simulink model "dodatkowa"  (R2022b)
settings: Solver=VariableStepAuto  StartTime=0.0  StopTime=10.0  RelTol=1e-3
values from neighbouring files (symbols this model uses):
  A = [0,       1,             0, 0 ... (first row only)    [dodatkowe.m]
  b = [0, 1/M, 0, 1/(M*L)]'    [dodatkowe.m]
  C = [1,0,0,0 ... (first row only)    [dodatkowe.m]
  D = [0, 0, 0,0]'    [dodatkowe.m]
  K = lqr(system, Q, R)    [dodatkowe.m]
  x0 = [0, 0, 0, 0]'    [dodatkowe.m]
  Y = [y, 0, 0, 0]'    [dodatkowe.m]
libraries: eeLuenbergerObserver x1
settings Model: Creator=student  LastModifiedBy=asialalala
settings SolverCC: AlgebraicLoopSolver=TrustRegion
settings OptimizationCC: ReuseModelBlockBuffer=on
settings DebuggingCC: UnconnectedInputMsg=warning  UnconnectedOutputMsg=warning  UnconnectedLineMsg=warning
settings ModelReferenceCC: EnableRefExpFcnMdlSchedulingChecks=on
settings RTWCC: DLArmComputeVersion=19.05

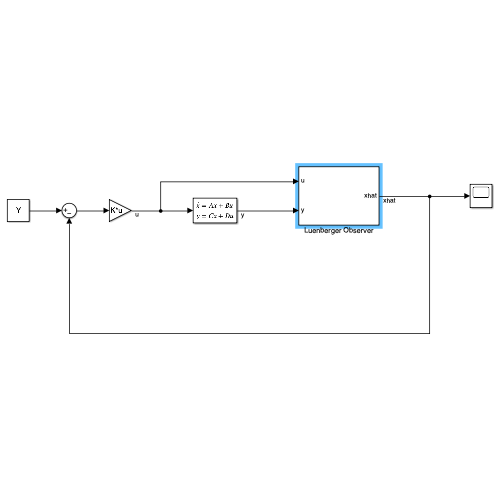
[thumbnail: Simulink's stored preview of the top-level diagram]
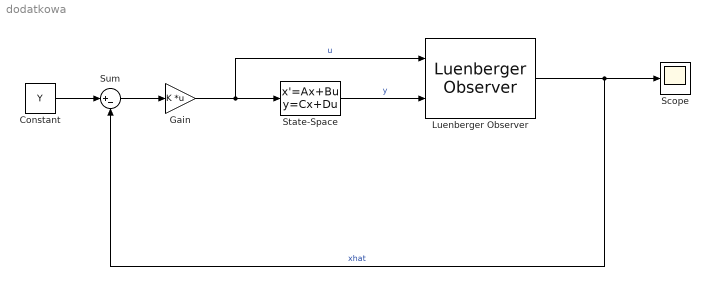
== system dodatkowa ==
  Constant : Constant  Value=Y
  Gain : Gain  Gain=K  Multiplication=Matrix(K*u)
  Luenberger Observer : eeLuenbergerObserver/Luenberger Observer  StateSpaceType=Continuous-time  Ad=A  Bd=b  Cd=C  Dd=D  A=A  B=b  C=C  D=D  ObserverDesign=Observer gain  Ld=2  DesiredEigenvalues=lambda  x0=x0  Tsd=0.1  Ts=0.001
  Scope : Scope
  State-Space : StateSpace  A=A  B=b  C=C  D=D  InitialCondition=x0
  Sum : Sum  Inputs=|+-
  wires:
  State-Space/1 -> Luenberger Observer/2  "y"
  Constant/1 -> Sum/1
  Sum/1 -> Gain/1
  Gain/1 -> Luenberger Observer/1, State-Space/1  "u"
  Luenberger Observer/1 -> Scope/1, Sum/2  "xhat"
